simulink model "pulse_detector_v1"  (R2022b)
settings: Solver=VariableStepAuto  StartTime=0.0  StopTime=SimTime  RelTol=1e-3
undefined symbols (not defined in the file): CorrFilter, threshold, WindowLen
libraries: simulink x1, dspsrcs4 x1, hdlsllib x1
settings Model: Creator=Lenovo  LastModifiedBy=Lenovo

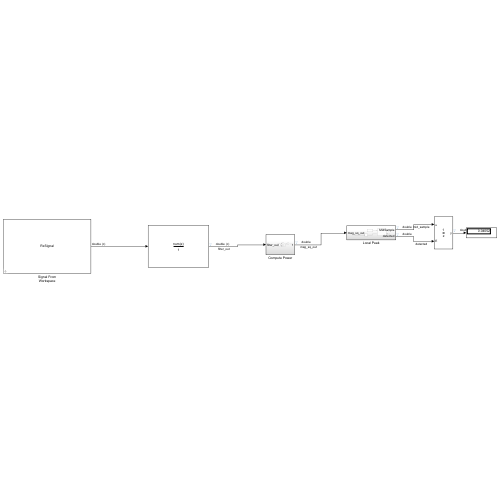
[thumbnail: Simulink's stored preview of the top-level diagram]
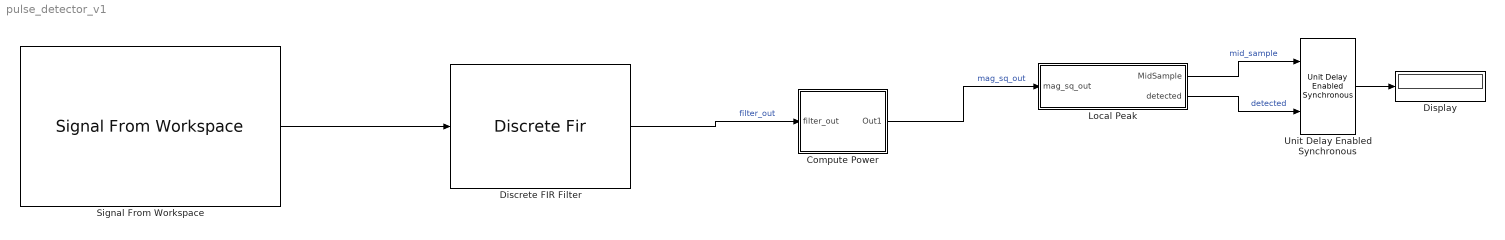
== system pulse_detector_v1 ==
  Compute Power : Subsystem
  Discrete FIR Filter : DiscreteFir  Coefficients=CorrFilter
  Display : Display
  Local Peak : Subsystem
  Signal From Workspace : dspsrcs4/Signal From Workspace  X=RxSignal  Ts=1  nsamps=1  OutputAfterFinalValue=Setting to zero  ignoreOrWarnInputAndFrameLengths=off  OutputFrames=off
  Unit Delay Enabled Synchronous : hdlsllib/Discrete/Unit Delay Enabled Synchronous  InitialCondition=0.0  SampleTime=-1
  wires:
  Signal From Workspace/1 -> Discrete FIR Filter/1
  Discrete FIR Filter/1 -> Compute Power/1(filter_out)  "filter_out"
  Compute Power/1(Out1) -> Local Peak/1(mag_sq_out)  "mag_sq_out"
  Local Peak/1(MidSample) -> Unit Delay Enabled Synchronous/1  "mid_sample"
  Local Peak/2(detected) -> Unit Delay Enabled Synchronous/2  "detected"
  Unit Delay Enabled Synchronous/1 -> Display/1

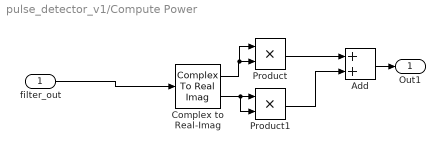
== system pulse_detector_v1/Compute Power ==
  filter_out : Inport
  Add : Sum
  Complex to Real-Imag : ComplexToRealImag
  Product : Product
  Product1 : Product
  Out1 : Outport
  wires:
  filter_out/1 -> Complex to Real-Imag/1
  Product/1 -> Add/1
  Complex to Real-Imag/2 -> Product1/2, Product1/1
  Complex to Real-Imag/1 -> Product/1, Product/2
  Product1/1 -> Add/2
  Add/1 -> Out1/1

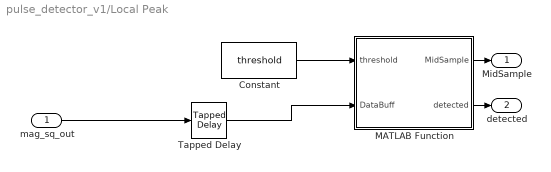
== system pulse_detector_v1/Local Peak ==
  mag_sq_out : Inport
  Constant : Constant  Value=threshold
  MATLAB Function : MATLAB Function  TreatAsAtomicUnit=on
  Tapped Delay : simulink/Discrete/Tapped Delay  vinit=0.0  samptime=-1  NumDelays=WindowLen  DelayOrder=Oldest  includeCurrent=off
  MidSample : Outport
  detected : Outport  Port=2
  wires:
  Constant/1 -> MATLAB Function/1(threshold)
  MATLAB Function/2(detected) -> detected/1
  Tapped Delay/1 -> MATLAB Function/2(DataBuff)
  MATLAB Function/1(MidSample) -> MidSample/1
  mag_sq_out/1 -> Tapped Delay/1

== matlab function pulse_detector_v1/Local Peak/MATLAB Function ==
  data: MidSample output; threshold input; DataBuff input; detected output; WindowLen parameter
function [MidSample,detected]=fcn(threshold,DataBuff, WindowLen)

MidIdx = ceil(WindowLen/2);

MidSample=DataBuff(MidIdx);
CompareOut=DataBuff-MidSample;



    % if all values in the result are negative and the middle sample is
    % greater than a threshold, it is a local max
if all(CompareOut <= 0) && (MidSample > threshold)
    detected=1;
else
    detected=0;
end
